simulink model "mdl_with_SMC"  (R2025b)
settings: Solver=FixedStepAuto  StartTime=0.0  StopTime=Tsim  FixedStep=Ts  RelTol=1e-3
values from neighbouring files (symbols this model uses):
  IC = [0,deg2rad(1),0,0]    [Copy_of_main_final.m]
  input_select = [1,0]    [Copy_of_main_final.m]
  phi = -x_cart / R    [animate_pendulum_cart_wheel_.m]
  plant_ss = plant_ss_q1    [Copy_of_main_final.m]    (also in syst_repr_generator.m = ss(A,B,C,D))
  plant_ss_diag = diagonalize(plant_ss)    [Copy_of_main_final.m]    (also in diagonalize.m = ss(A_d, B_d, C_d, 0))
  q2_f = deg2rad(10)    [Copy_of_main_final.m]
undefined symbols (not defined in the file or in its folder): alpha, F, k0, params
libraries: SignalEditorBlockLib x1
settings Model: Creator=dsagn  LastModifiedBy=dsagn
settings SolverCC: AlgebraicLoopSolver=TrustRegion
settings DataIOCC: ReturnWorkspaceOutputs=off
settings DebuggingCC: UnconnectedInputMsg=warning  UnconnectedOutputMsg=warning  UnconnectedLineMsg=warning  ArithmeticOperatorsInVariantConditions=warning
settings ModelReferenceCC: EnableRefExpFcnMdlSchedulingChecks=on
settings SFSimCC: CustomCodeUndefinedFunction=UseInterfaceOnly
settings RTWCC: GPUComputeCapability=3.5

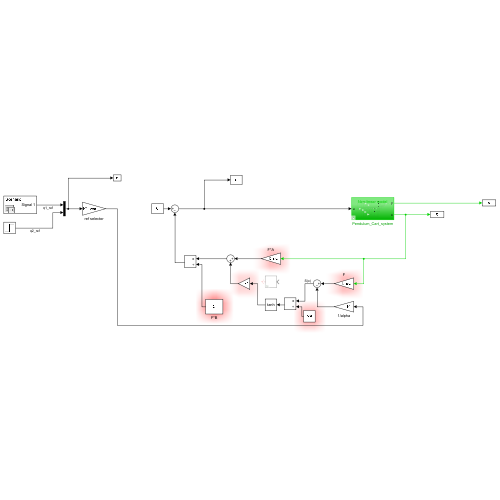
[thumbnail: Simulink's stored preview of the top-level diagram]
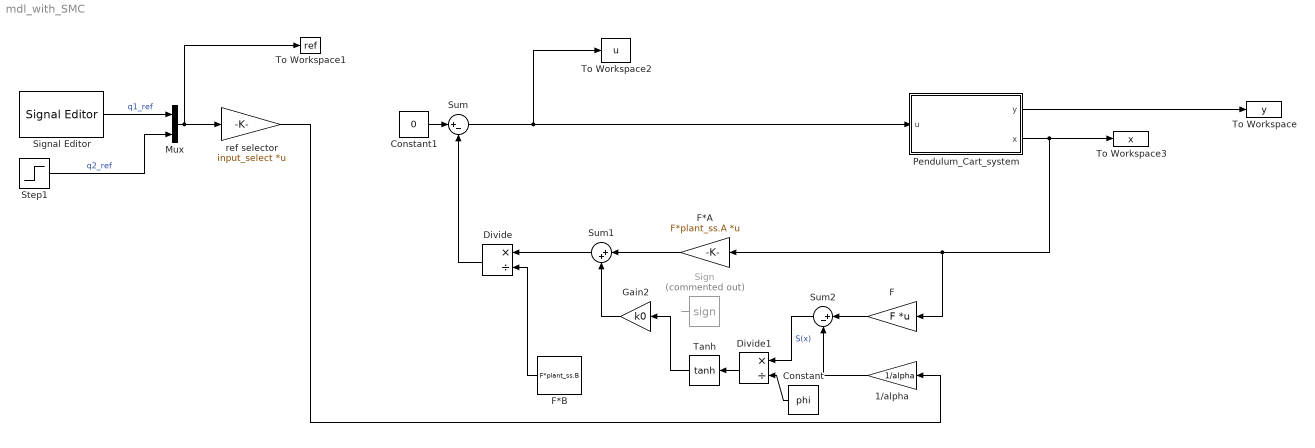
== system mdl_with_SMC ==
  1/alpha : Gain  Gain=1/alpha
  Constant : Constant  Value=phi
  Constant1 : Constant  Value=0
  Divide : Product  Inputs=*/
  Divide1 : Product  Inputs=*/
  F : Gain  Gain=F  Multiplication=Matrix(K*u) (u vector)
  F*A : Gain  Gain=F*plant_ss.A  Multiplication=Matrix(K*u) (u vector)
  F*B : Constant  Value=F*plant_ss.B
  Gain2 : Gain  Gain=k0
  Mux : Mux  Inputs=2
  Pendulum_Cart_system : Subsystem  Variant=on
  Sign : Signum  Commented=on
  Signal Editor : SignalEditorBlockLib/Signal Editor  FileName=q1_scenario1.mat  ActiveScenario=Scenario  ActiveSignal=Signal 1  IsBus=off  OutputBusObjectStr=Bus: BusObject  SampleTime=0  ZeroCross=off  OutputAfterFinalValue=Setting to zero  Unit=inherit  PreserveSignalName=on  ApplySigPropsToAllScenarios=on  ApplySigPropsToAllSignals=off  SignalPropertySource=Dialog parameters
  Step1 : Step  After=q2_f  SampleTime=0
  Sum : Sum  Inputs=|+-
  Sum1 : Sum  Inputs=|++
  Sum2 : Sum  Inputs=|+-
  Tanh : Trigonometry  Operator=tanh
  To Workspace : ToWorkspace  VariableName=y  SaveFormat=Timeseries  SampleTime=-1
  To Workspace1 : ToWorkspace  VariableName=ref  SaveFormat=Timeseries  SampleTime=-1
  To Workspace2 : ToWorkspace  VariableName=u  SaveFormat=Timeseries  SampleTime=-1
  To Workspace3 : ToWorkspace  VariableName=x  SaveFormat=Timeseries  SampleTime=-1
  ref selector : Gain  Gain=input_select  Multiplication=Matrix(K*u) (u vector)
  wires:
  ref selector/1 -> 1/alpha/1
  Pendulum_Cart_system/2(x) -> F*A/1, F/1, To Workspace3/1
  Pendulum_Cart_system/1(y) -> To Workspace/1
  Step1/1 -> Mux/2  "q2_ref"
  Mux/1 -> To Workspace1/1, ref selector/1
  Signal Editor/1 -> Mux/1  "q1_ref"
  Sum/1 -> To Workspace2/1, Pendulum_Cart_system/1(u)
  F*A/1 -> Sum1/1
  Gain2/1 -> Sum1/2
  Sign/1 -> ?
  Sum2/1 -> Divide1/1  "S(x)"
  Sum1/1 -> Divide/1
  F*B/1 -> Divide/2
  Divide/1 -> Sum/2
  Constant1/1 -> Sum/1
  F/1 -> Sum2/1
  1/alpha/1 -> Sum2/2
  Divide1/1 -> Tanh/1
  Constant/1 -> Divide1/2
  Tanh/1 -> Gain2/1

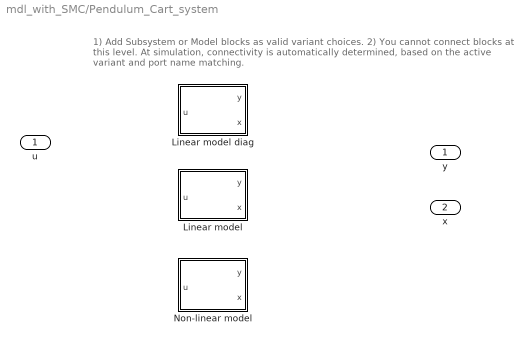
== system mdl_with_SMC/Pendulum_Cart_system ==
  note: 1) Add Subsystem or Model blocks as valid variant choices.
      | 2) You cannot connect blocks at this level. At simulation, connectivity is automatically
      | determined, based on the active variant and port name matching.
  u : Inport
  "Linear model " : Subsystem  VariantControl=model==1
  Linear model diag : Subsystem  VariantControl=model==2
  Non-linear model : Subsystem  VariantControl=model==3
  y : Outport
  x : Outport  Port=2

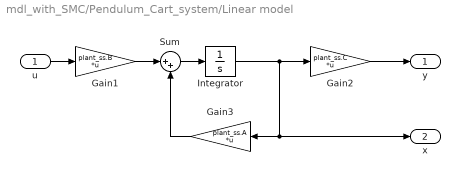
== system mdl_with_SMC/Pendulum_Cart_system/Linear model  ==
  u : Inport
  Gain1 : Gain  Gain=plant_ss.B  Multiplication=Matrix(K*u) (u vector)
  Gain2 : Gain  Gain=plant_ss.C  Multiplication=Matrix(K*u) (u vector)
  Gain3 : Gain  Gain=plant_ss.A  Multiplication=Matrix(K*u) (u vector)
  Integrator : Integrator  InitialCondition=IC
  Sum : Sum  Inputs=|++
  y : Outport
  x : Outport  Port=2
  wires:
  u/1 -> Gain1/1
  Gain1/1 -> Sum/1
  Sum/1 -> Integrator/1
  Gain3/1 -> Sum/2
  Integrator/1 -> Gain2/1, Gain3/1, x/1
  Gain2/1 -> y/1

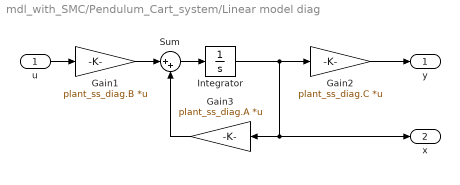
== system mdl_with_SMC/Pendulum_Cart_system/Linear model diag ==
  u : Inport
  Gain1 : Gain  Gain=plant_ss_diag.B  Multiplication=Matrix(K*u) (u vector)
  Gain2 : Gain  Gain=plant_ss_diag.C  Multiplication=Matrix(K*u) (u vector)
  Gain3 : Gain  Gain=plant_ss_diag.A  Multiplication=Matrix(K*u) (u vector)
  Integrator : Integrator  InitialCondition=IC
  Sum : Sum  Inputs=|++
  y : Outport
  x : Outport  Port=2
  wires:
  Gain2/1 -> y/1
  Integrator/1 -> x/1, Gain3/1, Gain2/1
  Gain3/1 -> Sum/2
  Sum/1 -> Integrator/1
  Gain1/1 -> Sum/1
  u/1 -> Gain1/1

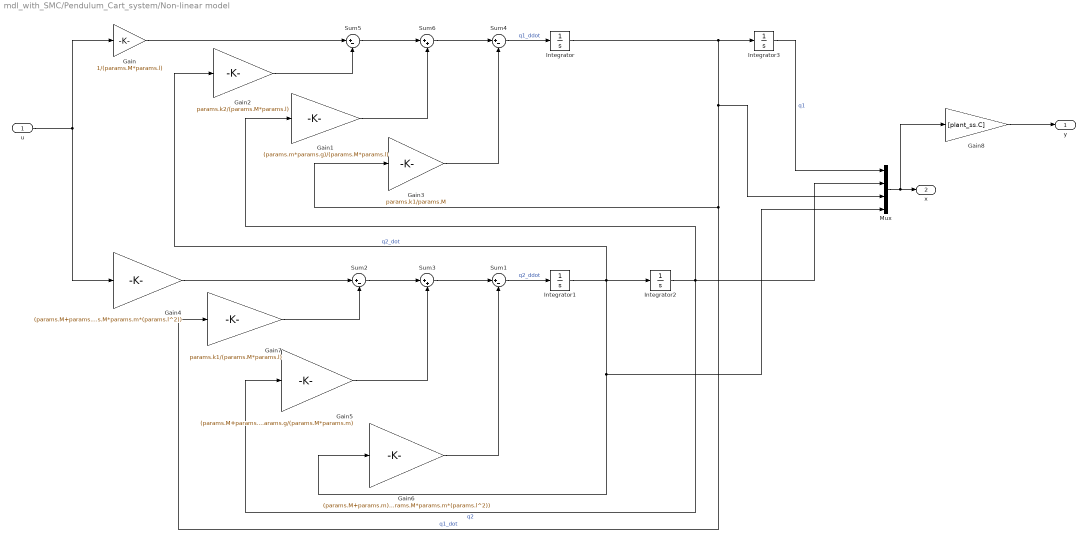
== system mdl_with_SMC/Pendulum_Cart_system/Non-linear model ==
  "u " : Inport
  Gain : Gain  Gain=1/(params.M*params.l)
  Gain1 : Gain  Gain=(params.m*params.g)/(params.M*params.l)
  Gain2 : Gain  Gain=params.k2/(params.M*params.l)
  Gain3 : Gain  Gain=params.k1/params.M
  Gain4 : Gain  Gain=(params.M+params.m)/(params.M*params.m*(params.l^2))
  Gain5 : Gain  Gain=(params.M+params.m)*params.g/(params.M*params.m)
  Gain6 : Gain  Gain=(params.M+params.m)*params.k2/(params.M*params.m*(params.l^2))
  Gain7 : Gain  Gain=params.k1/(params.M*params.l)
  Gain8 : Gain  Gain=[plant_ss.C]
  Integrator : Integrator
  Integrator1 : Integrator
  Integrator2 : Integrator  InitialCondition=IC(2)
  Integrator3 : Integrator
  Mux : Mux
  Sum{1..2,4..5} (4 alike) : Sum  Inputs=|+-
  Sum3 : Sum  Inputs=|++
  Sum6 : Sum  Inputs=|++
  y : Outport  VectorParamsAs1DForOutWhenUnconnected=off
  x : Outport  Port=2
  wires:
  Sum4/1 -> Integrator/1  "q1_ddot"
  "u "/1 -> Gain4/1, Gain/1
  Gain1/1 -> Sum6/2
  Gain2/1 -> Sum5/2
  Gain3/1 -> Sum4/2
  Integrator/1 -> Integrator3/1, Mux/3, Gain7/1, Gain3/1  "q1_dot"
  Gain4/1 -> Sum2/1
  Gain5/1 -> Sum3/2
  Gain6/1 -> Sum1/2
  Gain7/1 -> Sum2/2
  Sum1/1 -> Integrator1/1  "q2_ddot"
  Integrator1/1 -> Mux/4, Gain6/1, Gain2/1, Integrator2/1  "q2_dot"
  Integrator2/1 -> Mux/2, Gain5/1, Gain1/1  "q2"
  Sum2/1 -> Sum3/1
  Sum3/1 -> Sum1/1
  Sum6/1 -> Sum4/1
  Gain/1 -> Sum5/1
  Sum5/1 -> Sum6/1
  Integrator3/1 -> Mux/1  "q1"
  Mux/1 -> Gain8/1, x/1
  Gain8/1 -> y/1
